simulink model "H_Bridge_Converter_and_DC_Machine"  (R2021b)
settings: Solver=VariableStepAuto  StartTime=0.0  StopTime=8  MaxStep=T.FFT  RelTol=1e-3
undefined symbols (not defined in the file or in its folder): DC, omega_ref, T, torque_load
libraries: spsMosfetLib x4, spsVoltageMeasurementLib x3, spsControlledCurrentSourceLib x2, spsGroundLib x2, simulink x1, spsControlledVoltageSourceLib x1, spsCurrentMeasurementLib x1, spsDCVoltageSourceLib x1, spspowerguiLib x1
settings Model: Creator=junfei  LastModifiedBy=emmag
settings SolverCC: AlgebraicLoopSolver=TrustRegion
settings DataIOCC: SaveOutput=off  SignalLogging=off  DSMLogging=off  SaveTime=off  ReturnWorkspaceOutputs=off
settings DebuggingCC: UnconnectedInputMsg=none  UnconnectedOutputMsg=none  UnconnectedLineMsg=none  SFMachineParentedDataDiag=warning

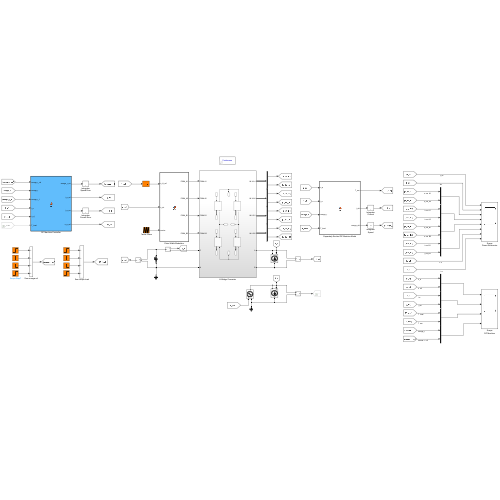
[thumbnail: Simulink's stored preview of the top-level diagram]
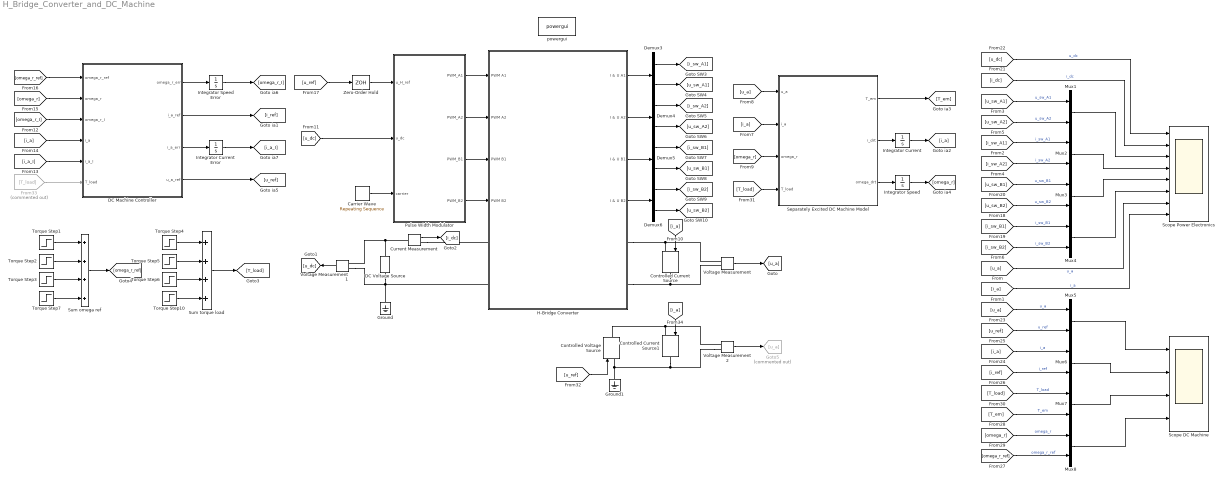
== system H_Bridge_Converter_and_DC_Machine ==
  Carrier Wave : simulink/Sources/Repeating Sequence  rep_seq_t=[0 T.sw/2 T.sw]  rep_seq_y=[-0.5 0.5 -0.5]
  Controlled Current Source : spsControlledCurrentSourceLib/Controlled Current Source  Initialize=off  Source_Type=DC  Amplitude=0  Phase=0  Frequency=0  Measurements=Current
  Controlled Current Source1 : spsControlledCurrentSourceLib/Controlled Current Source  Initialize=off  Source_Type=DC  Amplitude=0  Phase=0  Frequency=0  Measurements=Current
  Controlled Voltage Source : spsControlledVoltageSourceLib/Controlled Voltage Source  Initialize=off  Source_Type=DC  Amplitude=0  Phase=0  Frequency=0  Measurements=None
  Current Measurement : spsCurrentMeasurementLib/Current Measurement  PhasorSimulation=off  OutputType=Complex  PSBequivalent=0
  DC Machine Controller : MATLAB Function  TreatAsAtomicUnit=on
  DC Voltage Source : spsDCVoltageSourceLib/DC Voltage Source  Amplitude=DC.U  Measurements=Voltage
  Demux{3..6} (4 alike) : Demux  Outputs=2
  From33 : From  Commented=on  GotoTag=T_load
  Goto5 : Goto  Commented=on  GotoTag=u_a
  Ground : spsGroundLib/Ground  LConnTagsString=a
  Ground1 : spsGroundLib/Ground  LConnTagsString=a
  H-Bridge Converter : Subsystem
  Integrator Current : Integrator
  Integrator Current Error : Integrator
  Integrator Speed : Integrator
  Integrator Speed Error : Integrator
  Mux{1..8} (8 alike) : Mux  Inputs=2
  Pulse Width Modulator : MATLAB Function  TreatAsAtomicUnit=on
  Scope DC Machine : Scope  NumInputPorts=4
  Scope Power Electronics : Scope  NumInputPorts=8
  Separately Excited DC Machine Model : MATLAB Function  TreatAsAtomicUnit=on
  Sum omega ref : Sum  Inputs=++++
  Sum torque load : Sum  Inputs=++++
  Torque Step1 : Step  Time=omega_ref.time_1  After=omega_ref.step_1  SampleTime=0
  Torque Step10 : Step  Time=torque_load.time_4  After=torque_load.step_4  SampleTime=0
  Torque Step2 : Step  Time=omega_ref.time_2  After=omega_ref.step_2  SampleTime=0
  Torque Step3 : Step  Time=omega_ref.time_3  After=omega_ref.step_3  SampleTime=0
  Torque Step4 : Step  Time=torque_load.time_1  After=torque_load.step_1  SampleTime=0
  Torque Step5 : Step  Time=torque_load.time_2  After=torque_load.step_2  SampleTime=0
  Torque Step6 : Step  Time=torque_load.time_3  After=torque_load.step_3  SampleTime=0
  Torque Step7 : Step  Time=omega_ref.time_4  After=omega_ref.step_4  SampleTime=0
  Voltage Measurement : spsVoltageMeasurementLib/Voltage Measurement  PhasorSimulation=off  OutputType=Complex  PSBequivalent=0
  Voltage Measurement1 : spsVoltageMeasurementLib/Voltage Measurement  PhasorSimulation=off  OutputType=Complex  PSBequivalent=0
  Voltage Measurement2 : spsVoltageMeasurementLib/Voltage Measurement  PhasorSimulation=off  OutputType=Complex  PSBequivalent=0
  Zero-Order Hold : ZeroOrderHold  SampleTime=T.sw
  powergui : spspowerguiLib/powergui  Priority=1  SimulationMode=Continuous  SampleTime=50e-6  frequency=60  Iterations=50  frequencyindice=0  Pbase=100e6  ErrMax=1e-4  UnitsV=kV  UnitsW=MW  buscounter=0  FunctionMessages=off  echomessages=off  EnableUseOfTLC=off  CurrentSourceSwitches=off  DisableSnubberDevices=off  DisableRonSwitches=off  DisableVfSwitches=off  DisplayEquations=off  AutomaticDiscreteSolvers=off  SolverType=Tustin/Backward Euler (TBE)  Interpol=off  ExternalGateDelay=off  methode=off  Ts=100  x0status=blocks  SPID=on  SwTol=0  HookPort=off  NonlinearTolerance=1e-4  nMaxIteration=100  ContinueOnMaxIteration=off  RestoreLinks=warning  ResistiveCurrentMeasurement=off  Frange=[0:2:500]  Ylog=off  Xlog=on  ShowGrid=off  save=off  variable=ZData  structure=0  ZoomFFT=off  StartTime=0.0  cycles=1  DisplayStyle=1  fundamental=60  FreqAxis=off  MaxFrequency=1000  frequencyindicesteady=1  RmsSteady=1  display=off
  wires:
  Separately Excited DC Machine Model/3(omega_drt) -> Integrator Speed/1
  Separately Excited DC Machine Model/2(i_drt) -> Integrator Current/1
  Integrator Current/1 -> [i_a]
  [i_a] -> Separately Excited DC Machine Model/2(i_a)
  [u_a] -> Separately Excited DC Machine Model/1(u_a)
  Separately Excited DC Machine Model/1(T_em) -> [T_em]
  [T_load] -> Separately Excited DC Machine Model/4(T_load)
  Integrator Speed/1 -> [omega_r]
  [omega_r] -> Separately Excited DC Machine Model/3(omega_r)
  Pulse Width Modulator/1(PWM_A1) -> H-Bridge Converter/1(PWM A1)
  Pulse Width Modulator/2(PWM_A2) -> H-Bridge Converter/2(PWM A2)
  Pulse Width Modulator/3(PWM_B1) -> H-Bridge Converter/3(PWM B1)
  Pulse Width Modulator/4(PWM_B2) -> H-Bridge Converter/4(PWM B2)
  Carrier Wave/1 -> Pulse Width Modulator/3(carrier)
  Voltage Measurement1/1 -> [u_dc]
  [u_dc] -> Pulse Width Modulator/2(u_dc)
  Zero-Order Hold/1 -> Pulse Width Modulator/1(u_H_ref)
  DC Machine Controller/3(i_a_err) -> Integrator Current Error/1
  DC Machine Controller/1(omega_r_err) -> Integrator Speed Error/1
  DC Machine Controller/2(i_a_ref) -> [i_ref]
  DC Machine Controller/4(u_a_ref) -> [u_ref]
  Integrator Speed Error/1 -> [omega_r_I]
  Integrator Current Error/1 -> [i_a_I]
  [omega_r_I] -> DC Machine Controller/3(omega_r_I)
  [i_a_I] -> DC Machine Controller/5(i_a_I)
  [i_a] -> DC Machine Controller/4(i_a)
  [omega_r_ref] -> DC Machine Controller/1(omega_r_ref)
  [u_ref] -> Zero-Order Hold/1
  [omega_r] -> DC Machine Controller/2(omega_r)
  H-Bridge Converter/1(I & U A1) -> Demux3/1
  Demux3/1 -> [i_sw_A1]
  Demux3/2 -> [u_sw_A1]
  Demux4/1 -> [i_sw_A2]
  H-Bridge Converter/2(I & U A2) -> Demux4/1
  Demux4/2 -> [u_sw_A2]
  Demux5/1 -> [i_sw_B1]
  H-Bridge Converter/3(I & U B1) -> Demux5/1
  Demux5/2 -> [u_sw_B1]
  Demux6/1 -> [i_sw_B2]
  H-Bridge Converter/4(I & U B2) -> Demux6/1
  Demux6/2 -> [u_sw_B2]
  Current Measurement/1 -> [i_dc]
  [u_sw_A1] -> Mux1/1  "u_sw_A1"
  [u_sw_A2] -> Mux1/2  "u_sw_A2"
  [i_sw_A1] -> Mux2/1  "i_sw_A1"
  [i_sw_A2] -> Mux2/2  "i_sw_A2"
  [u_sw_B2] -> Mux3/2  "u_sw_B2"
  [i_sw_B1] -> Mux4/1  "i_sw_B1"
  [u_sw_B1] -> Mux3/1  "u_sw_B1"
  [i_sw_B2] -> Mux4/2  "i_sw_B2"
  [u_dc] -> Scope Power Electronics/1  "u_dc"
  [i_dc] -> Scope Power Electronics/2  "i_dc"
  Mux1/1 -> Scope Power Electronics/3
  Mux2/1 -> Scope Power Electronics/4
  Mux3/1 -> Scope Power Electronics/5
  Mux4/1 -> Scope Power Electronics/6
  [u_a] -> Scope Power Electronics/7  "u_a"
  [i_a] -> Scope Power Electronics/8  "i_a"
  Mux7/1 -> Scope DC Machine/3
  Mux8/1 -> Scope DC Machine/4
  Mux5/1 -> Scope DC Machine/1
  Mux6/1 -> Scope DC Machine/2
  Sum omega ref/1 -> [omega_r_ref]
  Sum torque load/1 -> [T_load]
  Torque Step2/1 -> Sum omega ref/2
  Torque Step3/1 -> Sum omega ref/3
  Torque Step4/1 -> Sum torque load/1
  Torque Step5/1 -> Sum torque load/2
  Torque Step6/1 -> Sum torque load/3
  Torque Step1/1 -> Sum omega ref/1
  Voltage Measurement/1 -> [u_a]
  [i_a] -> Controlled Current Source/1
  [u_ref] -> Controlled Voltage Source/1
  From33/1 -> DC Machine Controller/6(T_load)
  [i_a] -> Controlled Current Source1/1
  Voltage Measurement2/1 -> Goto5/1
  [u_a] -> Mux5/1  "u_a"
  [u_ref] -> Mux5/2  "u_ref"
  [i_a] -> Mux6/1  "i_a"
  [i_ref] -> Mux6/2  "i_ref"
  [T_load] -> Mux7/1  "T_load"
  [T_em] -> Mux7/2  "T_em"
  [omega_r] -> Mux8/1  "omega_r"
  [omega_r_ref] -> Mux8/2  "omega_r_ref"
  Torque Step7/1 -> Sum omega ref/4
  Torque Step10/1 -> Sum torque load/4
  connections:
  DC Voltage Source/RConn1 -- Current Measurement/LConn1 -- Voltage Measurement1/LConn1
  DC Voltage Source/LConn1 -- Ground/LConn1 -- H-Bridge Converter/LConn2 -- Voltage Measurement1/LConn2
  Current Measurement/RConn1 -- H-Bridge Converter/LConn1
  Voltage Measurement/LConn1 -- Controlled Current Source/LConn1 -- H-Bridge Converter/RConn1
  Voltage Measurement2/LConn2 -- Controlled Current Source1/RConn1 -- Ground1/LConn1 -- Controlled Voltage Source/LConn1
  Controlled Current Source/RConn1 -- H-Bridge Converter/RConn2 -- Voltage Measurement/LConn2
  Voltage Measurement2/LConn1 -- Controlled Voltage Source/RConn1 -- Controlled Current Source1/LConn1

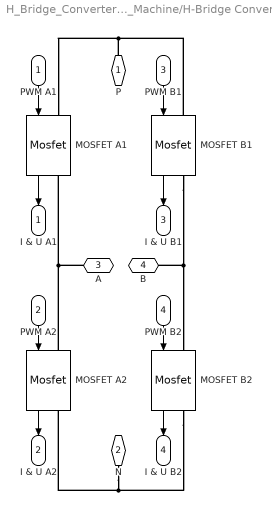
== system H_Bridge_Converter_and_DC_Machine/H-Bridge Converter ==
  PWM A1 : Inport
  PWM A2 : Inport  Port=2
  PWM B1 : Inport  Port=3
  PWM B2 : Inport  Port=4
  MOSFET A1 : spsMosfetLib/Mosfet  Ron=MOSFET.Ron  Lon=0  Rd=MOSFET.Rd  Vfd=MOSFET.Vf  IC=0  Rs=MOSFET.Rs  Cs=MOSFET.Cs  Measurements=on
  MOSFET A2 : spsMosfetLib/Mosfet  Ron=MOSFET.Ron  Lon=0  Rd=MOSFET.Rd  Vfd=MOSFET.Vf  IC=0  Rs=MOSFET.Rs  Cs=MOSFET.Cs  Measurements=on
  MOSFET B1 : spsMosfetLib/Mosfet  Ron=MOSFET.Ron  Lon=0  Rd=MOSFET.Rd  Vfd=MOSFET.Vf  IC=0  Rs=MOSFET.Rs  Cs=MOSFET.Cs  Measurements=on
  MOSFET B2 : spsMosfetLib/Mosfet  Ron=MOSFET.Ron  Lon=0  Rd=MOSFET.Rd  Vfd=MOSFET.Vf  IC=0  Rs=MOSFET.Rs  Cs=MOSFET.Cs  Measurements=on
  P : PMIOPort  Side=Left
  N : PMIOPort  Port=2  Side=Left
  A : PMIOPort  Port=3  Side=Right
  B : PMIOPort  Port=4  Side=Right
  I & U A1 : Outport
  I & U A2 : Outport  Port=2
  I & U B1 : Outport  Port=3
  I & U B2 : Outport  Port=4
  wires:
  PWM A1/1 -> MOSFET A1/1
  PWM B2/1 -> MOSFET B2/1
  PWM B1/1 -> MOSFET B1/1
  PWM A2/1 -> MOSFET A2/1
  MOSFET A1/1 -> I & U A1/1
  MOSFET B1/1 -> I & U B1/1
  MOSFET B2/1 -> I & U B2/1
  MOSFET A2/1 -> I & U A2/1
  connections:
  MOSFET B1/RConn1 -- MOSFET B2/LConn1 -- B/RConn1
  MOSFET A2/LConn1 -- MOSFET A1/RConn1 -- A/RConn1
  P/RConn1 -- MOSFET A1/LConn1 -- MOSFET B1/LConn1
  N/RConn1 -- MOSFET A2/RConn1 -- MOSFET B2/RConn1

== matlab function H_Bridge_Converter_and_DC_Machine/Pulse Width Modulator ==
  data: u_H_ref input; PWM_A1 output; u_dc input; carrier input; PWM_A2 output; PWM_B1 output; PWM_B2 output
function [PWM_A1,PWM_A2,PWM_B1,PWM_B2] = fcn(u_H_ref , u_dc , carrier)

duty_a_ref = + u_H_ref / 2 / u_dc;
duty_b_ref = - u_H_ref / 2 / u_dc;

PWM_A1 = duty_a_ref > carrier;
PWM_A2 = duty_a_ref < carrier;
PWM_B1 = duty_b_ref > carrier;
PWM_B2 = duty_b_ref < carrier;

end

== matlab function H_Bridge_Converter_and_DC_Machine/Separately Excited DC Machine Model ==
  data: u_a input; T_em output; i_a input; omega_r input; T_load input; i_drt output; omega_drt output; EM parameter
function [T_em, i_drt , omega_drt] = fcn(u_a , i_a , omega_r , T_load , EM)

i_drt = (u_a - EM.lambda * omega_r - EM.R_a * i_a) / EM.L_a;

T_em = EM.lambda * i_a;

omega_drt = (T_em - EM.B * omega_r - T_load) / EM.J;

end

== matlab function H_Bridge_Converter_and_DC_Machine/DC Machine Controller ==
  data: omega_r_ref input; omega_r_err output; omega_r input; omega_r_I input; i_a input; i_a_I input; T_load input; i_a_ref output; i_a_err output; u_a_ref output; ctrl parameter
function [omega_r_err , i_a_ref , i_a_err , u_a_ref] = fcn(omega_r_ref , omega_r , omega_r_I , i_a , i_a_I , T_load , ctrl)

% speed controller

omega_r_err = omega_r_ref - omega_r;

T_em_ref = ctrl.Kpw * omega_r_err + ctrl.Kiw * omega_r_I + T_load;

i_a_ref = T_em_ref / ctrl.lambda;

% current controller

i_a_err = i_a_ref - i_a;

u_a_ref = ctrl.Kpc * i_a_err + ctrl.Kic * i_a_I + ctrl.lambda * omega_r;

end
